simulink model "ES200A_CurrMeas"  (R2013b)
settings: Solver=FixedStepDiscrete  SolverMode=SingleTasking  StartTime=0.0  StopTime=1  FixedStep=0.000125  RelTol=1e-3
undefined symbols (not defined in the file): ARCHGLBPRM_2PI_ULS_F32, CurrMeasEolGainMax, CurrMeasEolGainMin, CurrMeasEolGainNrOfSample, CurrMeasEolGainNumer, CurrMeasEolMaxMotVel, CurrMeasEolOffsHiBrdgVltgMin, CurrMeasEolOffsHiCmuOffs, CurrMeasEolOffsLoCmuOffs, CurrMeasEolOffsMax, CurrMeasEolOffsMin, CurrMeasEolOffsNrOfSample, CurrMeasEolTranCntrThd, CurrMeasMinRqrdPhaOnTi, CurrMeasMotAgCompuDly, CurrMeasMotCurrAdcVlyWrmIninMax, CurrMeasMotCurrAdcVlyWrmIninMin, CurrMeasNtc0x05DFailStep, CurrMeasNtc0x05DPassStep, CurrMeasNtc0x06DFailStep, CurrMeasNtc0x06DPassStep, DEGREES30_MOTRAD_F32, DIFOFFSRNGCHKMAX_VOLT_F32, ELECGLBPRM_IVTRCNT_CNT_U08, ELECGLBPRM_STRTUPSTCURRMEASWRMININTESTSTRT_CNT_U08, FLTINJ_CURRMEAS_MOTCURRCORRDA, FLTINJ_CURRMEAS_MOTCURRCORRDD, FLTINJ_CURRMEAS_TESTOK, MAXCURRCORRD_AMPR_F32, PhaABCMeasdOutOfRng, PhaDEFMeasOutOfRng, SysGlbPrmMotPoleCnt
libraries: simulink x10, FixdToFloat x1
(part 3 of 7)

== system ES200A_CurrMeas/CurrMeas/CurrMeasGainWrReq ==
  CurrMeasMotCurrGainA_ArgIn : Inport  RequirementInfo={} %GIDa_c425d1ca_be7a_40e5_bba5_162e843ab10f  OutDataTypeStr=single
  CurrMeasMotCurrGainB_ArgIn : Inport  RequirementInfo={} %GIDa_bd7d1dd6_00d8_4c0e_b958_cd79b1c62016  Port=2  OutDataTypeStr=single
  CurrMeasMotCurrGainC_ArgIn : Inport  RequirementInfo={} %GIDa_442e802f_e2c7_406d_b1fc_b8f70d0353c6  Port=3  OutDataTypeStr=single
  CurrMeasMotCurrGainD_ArgIn : Inport  RequirementInfo={} %GIDa_a6de7fab_9a7f_4a18_932a_688a0ad19497  Port=4  OutDataTypeStr=single
  CurrMeasMotCurrGainE_ArgIn : Inport  RequirementInfo={} %GIDa_58241980_a2a0_46cb_8faf_4af881b5bc84  Port=5  OutDataTypeStr=single
  CurrMeasMotCurrGainF_ArgIn : Inport  RequirementInfo={} %GIDa_7c5d0880_7e38_46fb_95a6_ac4fe6cd7a27  Port=6  OutDataTypeStr=single
  function : TriggerPort
  Constant1 : Constant  Value=CurrMeasEolGainMax  OutDataTypeStr=single
  Constant3 : Constant  Value=CurrMeasEolGainMin  OutDataTypeStr=single
  CopyRight2 : Subsystem  Description=|  mask(Copyright Information){none=on}
      | Copyright info block.                                               
      |                                                                     
      | Place copyright information at the top of every subsystem in design.
      mask prompts: none "No parameters"
      mask help: Place copyright information at the top of every subsystem in design.
      mask Display:
      | NxtrConf = 'Nexteer Confidential';
      | 
      | sys = bdroot; %handle for the current model ("system")
      | first = get_param(sys,'Created');
      | first = first(end-3:end);  %year is last four digits
      | 
      | last = get_param(sys,'LastModifiedDate');
      | if isempty(last)
      |     last = datestr(now,'yyyy');
      | else
      |     last = last(end-3:end);
      | end
      | 
      | if strcmp(first,last)
      |     fprintf('%s -- Copyright %s Nexteer',NxtrConf,first)
      | else
      |     fprintf('%s -- %s%s- %s Nexteer',NxtrConf,char(169),first,last)
      | end
  IF : Subsystem  RequirementInfo={'linktype_rmi_doors' '000089bc (/ESG Group/FDD Module Requirements/EA4 Specific/ES200A_CurrMeas)' '#ES200A_291' 'true' 'REQ: ES200A_291' '' } %GIDa_4876ff6b_f5fc_4b95_bbc0_660fa9cc47c9  TreatAsAtomicUnit=on
  If1 : If  RequirementInfo={'linktype_rmi_doors' '000089bc (/ESG Group/FDD Module Requirements/EA4 Specific/ES200A_CurrMeas)' '#ES200A_291' 'true' 'REQ: ES200A_291' '' } %GIDa_99201fd8_db84_4d56_a868_77c34be46a9e  NumInputs=8  IfExpression=(u1 <= u3 & u3 <= u2) & (u1 <= u4 & u4 <= u2) & (u1 <= u5 & u5 <= u2) & (u1 <= u6 & u6 <= u2) & (u1 <= u7 & u7 <= u2) & (u1 <= u8 & u8 <= u2)
  Merge : Merge
  "else " : Subsystem  TreatAsAtomicUnit=on
  CurrMeasGainWrReqSts : Outport  RequirementInfo={} %GIDa_00298d30_c602_4e54_ac9c_fe9e46cb7e08
  wires:
  If1/1 -> IF/Action
  Constant3/1 -> If1/1
  Constant1/1 -> If1/2
  CurrMeasMotCurrGainC_ArgIn/1 -> IF/3(CurrMeasMotCurrGainC_ArgIn), If1/5  "CurrMeasMotCurrGainC_ArgIn"
  CurrMeasMotCurrGainD_ArgIn/1 -> IF/4(CurrMeasMotCurrGainD_ArgIn), If1/6  "CurrMeasMotCurrGainD_ArgIn"
  CurrMeasMotCurrGainB_ArgIn/1 -> IF/2(CurrMeasMotCurrGainB_ArgIn), If1/4  "CurrMeasMotCurrGainB_ArgIn"
  CurrMeasMotCurrGainE_ArgIn/1 -> IF/5(CurrMeasMotCurrGainE_ArgIn), If1/7  "CurrMeasMotCurrGainE_ArgIn"
  CurrMeasMotCurrGainA_ArgIn/1 -> IF/1(CurrMeasMotCurrGainA_ArgIn), If1/3  "CurrMeasMotCurrGainA_ArgIn"
  CurrMeasMotCurrGainF_ArgIn/1 -> IF/6(CurrMeasMotCurrGainF_ArgIn), If1/8  "CurrMeasMotCurrGainF_ArgIn"
  If1/2 -> "else "/Action
  Merge/1 -> CurrMeasGainWrReqSts/1
  "else "/1(CurrMeasGainWrReqSts) -> Merge/1
  IF/1(CurrMeasGainWrReqSts) -> Merge/2

== system ES200A_CurrMeas/CurrMeas/CurrMeasInit1 ==
  CurrMeasEolOffsHiBrdgVltgMin : Inport
  Trigger : TriggerPort  TriggerType=function-call  PortDimensions=1
  CopyRight2 : Subsystem  Description=|  mask(Copyright Information){none=on}
      | Copyright info block.                                               
      |                                                                     
      | Place copyright information at the top of every subsystem in design.
      mask prompts: none "No parameters"
      mask help: Place copyright information at the top of every subsystem in design.
      mask Display:
      | NxtrConf = 'Nexteer Confidential';
      | 
      | sys = bdroot; %handle for the current model ("system")
      | first = get_param(sys,'Created');
      | first = first(end-3:end);  %year is last four digits
      | 
      | last = get_param(sys,'LastModifiedDate');
      | if isempty(last)
      |     last = datestr(now,'yyyy');
      | else
      |     last = last(end-3:end);
      | end
      | 
      | if strcmp(first,last)
      |     fprintf('%s -- Copyright %s Nexteer',NxtrConf,first)
      | else
      |     fprintf('%s -- %s%s- %s Nexteer',NxtrConf,char(169),first,last)
      | end
  CurrMeasEolOffsCalSet : DataStoreRead  RequirementInfo={'linktype_rmi_doors' '000089bc (/ESG Group/FDD Module Requirements/EA4 Specific/ES200A_CurrMeas)' '#ES200A_280' 'true' 'REQ: ES200A_280' '' } %GIDa_5b13b3a8_fa13_45cc_ae87_baf34a1014a6  DataStoreName=CurrMeasEolOffsCalSet  DataStoreElements=CurrMeasEolOffsCalSet.CurrMeasMotCurrEolOffsDifA#CurrMeasEolOffsCalSet.CurrMeasMotCurrEolOffsDifB#CurrMeasEolOffsCalSet.CurrMeasMotCurrEolOffsDifC#CurrMeasEolOffsCalSet.CurrMeasEolOffsHiBrdgVltg#CurrMeasEolOffsCalSet.CurrMeasMotCurrEolOffsDifD#CurrMeasEolOffsCalSet.CurrMeasMotCurrEolOffsDifE#CurrMeasEolOffsCalSet.CurrMeasMotCurrEolOffsDifF
  If : If  NumInputs=2  IfExpression=u1>u2
  If Action Subsystem : Subsystem  TreatAsAtomicUnit=on
  If Action Subsystem1 : Subsystem  TreatAsAtomicUnit=on
  Merge{1..6} (6 alike) : Merge
  MotCurrOffsDeltaA : Outport
  MotCurrOffsDeltaB : Outport  Port=2
  MotCurrOffsDeltaC : Outport  Port=3
  MotCurrOffsDeltaD : Outport  Port=4
  MotCurrOffsDeltaE : Outport  Port=5
  MotCurrOffsDeltaF : Outport  Port=6
  wires:
  CurrMeasEolOffsHiBrdgVltgMin/1 -> If/2
  If/1 -> If Action Subsystem/Action
  If/2 -> If Action Subsystem1/Action
  If Action Subsystem/1(MotCurrOffsDeltaA) -> Merge1/1
  If Action Subsystem/2(MotCurrOffsDeltaB) -> Merge2/1
  If Action Subsystem/3(MotCurrOffsDeltaC) -> Merge3/1
  If Action Subsystem/4(MotCurrOffsDeltaD) -> Merge4/1
  If Action Subsystem/5(MotCurrOffsDeltaE) -> Merge5/1
  If Action Subsystem/6(MotCurrOffsDeltaF) -> Merge6/1
  If Action Subsystem1/1(MotCurrOffsDeltaA) -> Merge1/2
  If Action Subsystem1/2(MotCurrOffsDeltaB) -> Merge2/2
  If Action Subsystem1/3(MotCurrOffsDeltaC) -> Merge3/2
  If Action Subsystem1/4(MotCurrOffsDeltaD) -> Merge4/2
  If Action Subsystem1/5(MotCurrOffsDeltaE) -> Merge5/2
  If Action Subsystem1/6(MotCurrOffsDeltaF) -> Merge6/2
  Merge1/1 -> MotCurrOffsDeltaA/1
  Merge2/1 -> MotCurrOffsDeltaB/1
  Merge3/1 -> MotCurrOffsDeltaC/1
  Merge4/1 -> MotCurrOffsDeltaD/1
  Merge5/1 -> MotCurrOffsDeltaE/1
  Merge6/1 -> MotCurrOffsDeltaF/1
  CurrMeasEolOffsCalSet/5 -> If Action Subsystem/5(MotCurrEolOffsDifD)
  CurrMeasEolOffsCalSet/3 -> If Action Subsystem/3(MotCurrEolOffsDifC)
  CurrMeasEolOffsCalSet/6 -> If Action Subsystem/6(MotCurrEolOffsDifE)
  CurrMeasEolOffsCalSet/1 -> If Action Subsystem/1(MotCurrEolOffsDifA)
  CurrMeasEolOffsCalSet/2 -> If Action Subsystem/2(MotCurrEolOffsDifB)
  CurrMeasEolOffsCalSet/7 -> If Action Subsystem/7(MotCurrEolOffsDifF)
  CurrMeasEolOffsCalSet/4 -> If/1, If Action Subsystem/4(CurrMeasEolOffsHiBrdgVltg)

== system ES200A_CurrMeas/CurrMeas/CurrMeasOffsReadReq ==
  function : TriggerPort
  CopyRight2 : Subsystem  Description=|  mask(Copyright Information){none=on}
      | Copyright info block.                                               
      |                                                                     
      | Place copyright information at the top of every subsystem in design.
      mask prompts: none "No parameters"
      mask help: Place copyright information at the top of every subsystem in design.
      mask Display:
      | NxtrConf = 'Nexteer Confidential';
      | 
      | sys = bdroot; %handle for the current model ("system")
      | first = get_param(sys,'Created');
      | first = first(end-3:end);  %year is last four digits
      | 
      | last = get_param(sys,'LastModifiedDate');
      | if isempty(last)
      |     last = datestr(now,'yyyy');
      | else
      |     last = last(end-3:end);
      | end
      | 
      | if strcmp(first,last)
      |     fprintf('%s -- Copyright %s Nexteer',NxtrConf,first)
      | else
      |     fprintf('%s -- %s%s- %s Nexteer',NxtrConf,char(169),first,last)
      | end
  CurrMeasEolOffsCalSet : DataStoreRead  RequirementInfo={'linktype_rmi_doors' '000089bc (/ESG Group/FDD Module Requirements/EA4 Specific/ES200A_CurrMeas)' '#ES200A_280' 'true' 'REQ: ES200A_280' '' } %GIDa_8cba0bc8_e323_4e1f_8e86_73dafe0bba1d  DataStoreName=CurrMeasEolOffsCalSet  DataStoreElements=CurrMeasEolOffsCalSet.CurrMeasEolOffsHiBrdgVltg#CurrMeasEolOffsCalSet.CurrMeasMotCurrEolOffsDifA#CurrMeasEolOffsCalSet.CurrMeasMotCurrEolOffsDifB#CurrMeasEolOffsCalSet.CurrMeasMotCurrEolOffsDifC#CurrMeasEolOffsCalSet.CurrMeasMotCurrEolOffsDifD#CurrMeasEolOffsCalSet.CurrMeasMotCurrEolOffsDifE#CurrMeasEolOffsCalSet.CurrMeasMotCurrEolOffsDifF#CurrMeasEolOffsCalSet.CurrMeasMotCurrOffsLoAvrgA#CurrMeasEolOffsCalSet.CurrMeasMotCurrOffsLoAvrgB#CurrMeasEolOffsCalSet.CurrMeasMotCurrOffsLoAvrgC#CurrMeasEolOffsCalSet.CurrMeasMotCurrOffsLoAvrgD#CurrMeasEolOffsCalSet.CurrMeasMotCurrOffsLoAvrgE#CurrMeasEolOffsCalSet.CurrMeasMotCurrOffsLoAvrgF
  CurrMeasEolOffsHiBrdgVltg_ArgOut : Outport  RequirementInfo={} %GIDa_c2b0fe9d_3793_43b9_8623_9e15e29718c9
  CurrMeasMotCurrOffsDifA_ArgOut : Outport  RequirementInfo={} %GIDa_06880cd0_b3c9_4dac_a20b_1d769ce6ab3e  Port=2
  CurrMeasMotCurrOffsDifB_ArgOut : Outport  RequirementInfo={} %GIDa_89879a61_0bc4_4d01_9a03_1b0943ab4d4d  Port=3
  CurrMeasMotCurrOffsDifC_ArgOut : Outport  RequirementInfo={} %GIDa_a1432bf3_c07e_4e99_b270_4232122d4772  Port=4
  CurrMeasMotCurrOffsDifD_ArgOut : Outport  RequirementInfo={} %GIDa_3df17fd6_11a6_4a3b_a21f_0f2b4386103a  Port=5
  CurrMeasMotCurrOffsDifE_ArgOut : Outport  RequirementInfo={} %GIDa_8531bc1c_851e_4a5c_bd1a_ff758ac49903  Port=6
  CurrMeasMotCurrOffsDifF_ArgOut : Outport  RequirementInfo={} %GIDa_d9d2e87e_a616_4443_9719_46d0ee8ea0d2  Port=7
  CurrMeasMotCurrOffsLoAvrgA_ArgOut : Outport  RequirementInfo={} %GIDa_c5194a62_6435_4295_b125_fb72e5f95c25  Port=8
  CurrMeasMotCurrOffsLoAvrgB_ArgOut : Outport  RequirementInfo={} %GIDa_76f08b3f_5cc7_46f2_a183_091f4f2205e6  Port=9
  CurrMeasMotCurrOffsLoAvrgC_ArgOut : Outport  RequirementInfo={} %GIDa_b1bbc18a_9d6a_4672_bdc3_0bccd18a5fef  Port=10
  CurrMeasMotCurrOffsLoAvrgD_ArgOut : Outport  RequirementInfo={} %GIDa_3f8d0b0a_e576_41bf_81a1_80b77bc69872  Port=11
  CurrMeasMotCurrOffsLoAvrgE_ArgOut : Outport  RequirementInfo={} %GIDa_06d47c59_3406_4ddb_96f7_958a6ee8ee04  Port=12
  CurrMeasMotCurrOffsLoAvrgF_ArgOut : Outport  RequirementInfo={} %GIDa_8b869263_e1b4_42a0_8921_d65f6bf7b80b  Port=13
  wires:
  CurrMeasEolOffsCalSet/1 -> CurrMeasEolOffsHiBrdgVltg_ArgOut/1
  CurrMeasEolOffsCalSet/2 -> CurrMeasMotCurrOffsDifA_ArgOut/1
  CurrMeasEolOffsCalSet/3 -> CurrMeasMotCurrOffsDifB_ArgOut/1
  CurrMeasEolOffsCalSet/4 -> CurrMeasMotCurrOffsDifC_ArgOut/1
  CurrMeasEolOffsCalSet/5 -> CurrMeasMotCurrOffsDifD_ArgOut/1
  CurrMeasEolOffsCalSet/6 -> CurrMeasMotCurrOffsDifE_ArgOut/1
  CurrMeasEolOffsCalSet/7 -> CurrMeasMotCurrOffsDifF_ArgOut/1
  CurrMeasEolOffsCalSet/8 -> CurrMeasMotCurrOffsLoAvrgA_ArgOut/1
  CurrMeasEolOffsCalSet/9 -> CurrMeasMotCurrOffsLoAvrgB_ArgOut/1
  CurrMeasEolOffsCalSet/10 -> CurrMeasMotCurrOffsLoAvrgC_ArgOut/1
  CurrMeasEolOffsCalSet/11 -> CurrMeasMotCurrOffsLoAvrgD_ArgOut/1
  CurrMeasEolOffsCalSet/12 -> CurrMeasMotCurrOffsLoAvrgE_ArgOut/1
  CurrMeasEolOffsCalSet/13 -> CurrMeasMotCurrOffsLoAvrgF_ArgOut/1

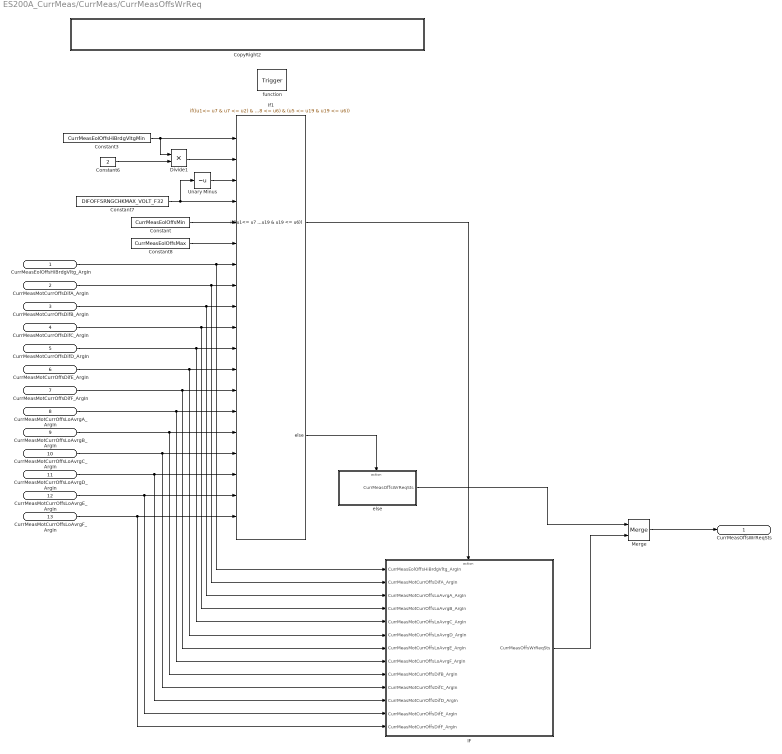
== system ES200A_CurrMeas/CurrMeas/CurrMeasOffsWrReq ==
  CurrMeasEolOffsHiBrdgVltg_ArgIn : Inport  RequirementInfo={} %GIDa_20319714_70ba_40b8_83d5_5be49dcbe6c0  OutDataTypeStr=single
  CurrMeasMotCurrOffsDifA_ArgIn : Inport  RequirementInfo={} %GIDa_567da3a1_0d48_4934_8feb_e936b086fb7e  Port=2  OutDataTypeStr=single
  CurrMeasMotCurrOffsDifB_ArgIn : Inport  RequirementInfo={} %GIDa_d0ed0aa3_f35f_4142_b108_d1399608bd37  Port=3  OutDataTypeStr=single
  CurrMeasMotCurrOffsDifC_ArgIn : Inport  RequirementInfo={} %GIDa_333f9d57_9630_4d9a_bf0a_758004fd24d5  Port=4  OutDataTypeStr=single
  CurrMeasMotCurrOffsDifD_ArgIn : Inport  RequirementInfo={} %GIDa_75702a95_bde2_4d36_99b5_54163b4c7153  Port=5  OutDataTypeStr=single
  CurrMeasMotCurrOffsDifE_ArgIn : Inport  RequirementInfo={} %GIDa_d5c11ab6_7fa1_4a01_9aa2_8e70eb92dca0  Port=6  OutDataTypeStr=single
  CurrMeasMotCurrOffsDifF_ArgIn : Inport  RequirementInfo={} %GIDa_93b2894a_d1d3_46df_b4ef_6d97a088df41  Port=7  OutDataTypeStr=single
  CurrMeasMotCurrOffsLoAvrgA_ArgIn : Inport  RequirementInfo={} %GIDa_d3fc1696_9b01_4bfe_ae5b_43ed0baf9797  Port=8  OutDataTypeStr=single
  CurrMeasMotCurrOffsLoAvrgB_ArgIn : Inport  RequirementInfo={} %GIDa_e3286a61_69ab_4ddc_b4c3_7297f20485dd  Port=9  OutDataTypeStr=single
  CurrMeasMotCurrOffsLoAvrgC_ArgIn : Inport  RequirementInfo={} %GIDa_d0fb0236_0795_4629_a145_caa3ab5bd346  Port=10  OutDataTypeStr=single
  CurrMeasMotCurrOffsLoAvrgD_ArgIn : Inport  RequirementInfo={} %GIDa_8377999d_f727_4278_a09a_19b59b7325e4  Port=11  OutDataTypeStr=single
  CurrMeasMotCurrOffsLoAvrgE_ArgIn : Inport  RequirementInfo={} %GIDa_308508b2_c858_4477_ae29_a4055a9a0165  Port=12  OutDataTypeStr=single
  CurrMeasMotCurrOffsLoAvrgF_ArgIn : Inport  RequirementInfo={} %GIDa_00179445_133e_4a7c_829d_b4552183115d  Port=13  OutDataTypeStr=single
  function : TriggerPort
  Constant : Constant  Value=CurrMeasEolOffsMin
  Constant3 : Constant  Value=CurrMeasEolOffsHiBrdgVltgMin  OutDataTypeStr=single
  Constant6 : Constant  Value=2  OutDataTypeStr=single
  Constant7 : Constant  Value=DIFOFFSRNGCHKMAX_VOLT_F32  OutDataTypeStr=single
  Constant8 : Constant  Value=CurrMeasEolOffsMax
  CopyRight2 : Subsystem  Description=|  mask(Copyright Information){none=on}
      | Copyright info block.                                               
      |                                                                     
      | Place copyright information at the top of every subsystem in design.
      mask prompts: none "No parameters"
      mask help: Place copyright information at the top of every subsystem in design.
      mask Display:
      | NxtrConf = 'Nexteer Confidential';
      | 
      | sys = bdroot; %handle for the current model ("system")
      | first = get_param(sys,'Created');
      | first = first(end-3:end);  %year is last four digits
      | 
      | last = get_param(sys,'LastModifiedDate');
      | if isempty(last)
      |     last = datestr(now,'yyyy');
      | else
      |     last = last(end-3:end);
      | end
      | 
      | if strcmp(first,last)
      |     fprintf('%s -- Copyright %s Nexteer',NxtrConf,first)
      | else
      |     fprintf('%s -- %s%s- %s Nexteer',NxtrConf,char(169),first,last)
      | end
  Divide1 : Product  Inputs=**  OutDataTypeStr=single
  IF : Subsystem  RequirementInfo={'linktype_rmi_doors' '000089bc (/ESG Group/FDD Module Requirements/EA4 Specific/ES200A_CurrMeas)' '#ES200A_280' 'true' 'REQ: ES200A_280' '' } %GIDa_94ca970e_96f2_476d_8160_5cb99576e311  TreatAsAtomicUnit=on
  If1 : If  RequirementInfo={'linktype_rmi_doors' '000089bc (/ESG Group/FDD Module Requirements/EA4 Specific/ES200A_CurrMeas)' '#ES200A_280' 'true' 'REQ: ES200A_280' '' } %GIDa_9a24cfae_c3f3_4b93_a488_aa733d7ab090  NumInputs=19  IfExpression=(u1<= u7 & u7 <= u2) & (u3 <= u8 & u8 <= u4) & (u3 <= u9 & u9 <= u4) & (u3 <= u10 & u10 < u4) & (u3 <= u11 & u11 <= u4) & (u3 <= u12 & u12 <= u4) & (u3 <= u13 & u13 <= u4) & (u5 <= u14 & u14 <= u6) & (u5 <= u15 & u15 <= u6) & (u5 <= u16 & u16 <= u6) & (u5 <= u17 & u17 <= u6) & (u5 <= u18 & u18 <= u6) & (u5 <= u19 & u19 <= u6)
  Merge : Merge
  Unary Minus : UnaryMinus
  "else " : Subsystem  TreatAsAtomicUnit=on
  CurrMeasOffsWrReqSts : Outport  RequirementInfo={} %GIDa_e38a5dae_03c2_4788_8854_754d30bf24dd
  wires:
  Constant3/1 -> If1/1, Divide1/1
  Constant6/1 -> Divide1/2
  Unary Minus/1 -> If1/3
  Constant7/1 -> Unary Minus/1, If1/4
  Constant8/1 -> If1/6
  Constant/1 -> If1/5
  CurrMeasEolOffsHiBrdgVltg_ArgIn/1 -> IF/1(CurrMeasEolOffsHiBrdgVltg_ArgIn), If1/7
  CurrMeasMotCurrOffsDifA_ArgIn/1 -> IF/2(CurrMeasMotCurrOffsDifA_ArgIn), If1/8
  CurrMeasMotCurrOffsDifB_ArgIn/1 -> IF/3(CurrMeasMotCurrOffsLoAvrgA_ArgIn), If1/9
  CurrMeasMotCurrOffsDifC_ArgIn/1 -> IF/4(CurrMeasMotCurrOffsLoAvrgB_ArgIn), If1/10
  CurrMeasMotCurrOffsDifD_ArgIn/1 -> IF/5(CurrMeasMotCurrOffsLoAvrgC_ArgIn), If1/11
  CurrMeasMotCurrOffsDifE_ArgIn/1 -> IF/6(CurrMeasMotCurrOffsLoAvrgD_ArgIn), If1/12
  CurrMeasMotCurrOffsLoAvrgA_ArgIn/1 -> IF/8(CurrMeasMotCurrOffsLoAvrgF_ArgIn), If1/14
  CurrMeasMotCurrOffsLoAvrgB_ArgIn/1 -> IF/9(CurrMeasMotCurrOffsDifB_ArgIn), If1/15
  CurrMeasMotCurrOffsLoAvrgE_ArgIn/1 -> IF/12(CurrMeasMotCurrOffsDifE_ArgIn), If1/18
  CurrMeasMotCurrOffsLoAvrgF_ArgIn/1 -> IF/13(CurrMeasMotCurrOffsDifF_ArgIn), If1/19
  CurrMeasMotCurrOffsLoAvrgC_ArgIn/1 -> IF/10(CurrMeasMotCurrOffsDifC_ArgIn), If1/16
  If1/1 -> IF/Action
  CurrMeasMotCurrOffsDifF_ArgIn/1 -> IF/7(CurrMeasMotCurrOffsLoAvrgE_ArgIn), If1/13
  CurrMeasMotCurrOffsLoAvrgD_ArgIn/1 -> IF/11(CurrMeasMotCurrOffsDifD_ArgIn), If1/17
  If1/2 -> "else "/Action
  Divide1/1 -> If1/2
  Merge/1 -> CurrMeasOffsWrReqSts/1
  "else "/1(CurrMeasOffsWrReqSts) -> Merge/1
  IF/1(CurrMeasOffsWrReqSts) -> Merge/2

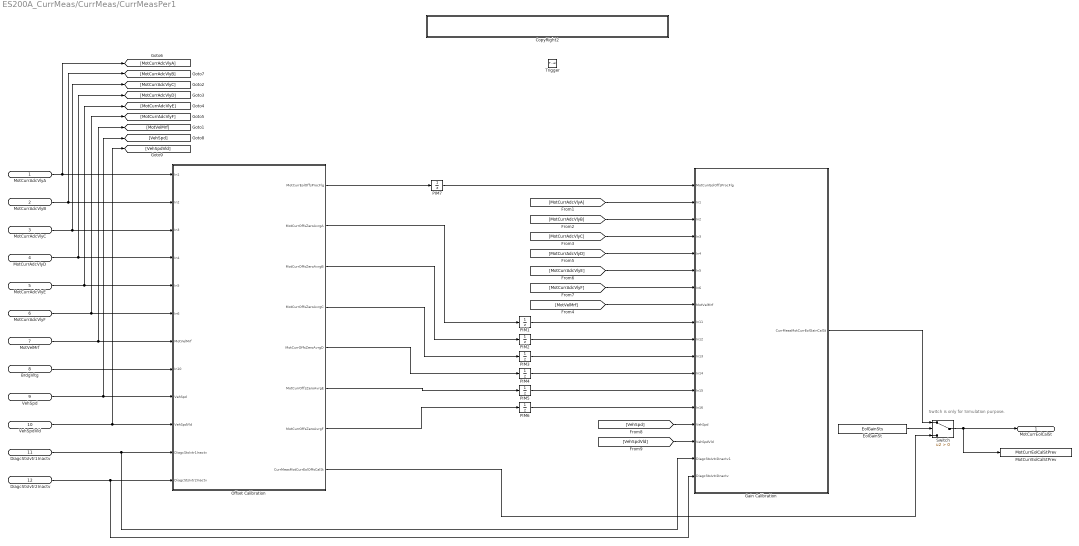
== system ES200A_CurrMeas/CurrMeas/CurrMeasPer1 ==
  note: Switch is only for Simulation purpose.
  MotCurrAdcVlyA : Inport  RequirementInfo={} %GIDa_d6fdc2a5_c36f_4862_a3e7_4b336023a3c4  OutDataTypeStr=single
  MotCurrAdcVlyB : Inport  RequirementInfo={} %GIDa_329e32be_6008_45fd_bd72_340d7ae8c1b5  Port=2  OutDataTypeStr=single
  MotCurrAdcVlyC : Inport  RequirementInfo={} %GIDa_746c9616_e976_40d7_b54a_823dc364fe71  Port=3  OutDataTypeStr=single
  MotCurrAdcVlyD : Inport  RequirementInfo={} %GIDa_4b06763f_6209_4b7f_9565_5c5d2daca03a  Port=4  OutDataTypeStr=single
  MotCurrAdcVlyE : Inport  RequirementInfo={} %GIDa_3a5b9e65_aa66_45a4_8818_13580434b978  Port=5  OutDataTypeStr=single
  MotCurrAdcVlyF : Inport  RequirementInfo={} %GIDa_3a4efe1c_5ef6_4746_95ad_6493d8eca6d1  Port=6  OutDataTypeStr=single
  MotVelMrf : Inport  RequirementInfo={} %GIDa_3549e207_a5ba_4370_a041_76429f88a9dd  Port=7  OutDataTypeStr=single
  BrdgVltg : Inport  RequirementInfo={} %GIDa_3ee59834_071a_42af_a764_5aee71a021cf  Port=8  OutDataTypeStr=single
  VehSpd : Inport  RequirementInfo={} %GIDa_3dad792b_6867_498d_8cf5_08b87633e71b  Port=9
  VehSpdVld : Inport  RequirementInfo={} %GIDa_79ad4a0e_1634_487e_a0d4_030cd7a6c3f9  Port=10
  DiagcStsIvtr1Inactv : Inport  RequirementInfo={} %GIDa_c8c114ff_24fe_44c5_88f9_1823b0535249  Port=11
  DiagcStsIvtr2Inactv : Inport  RequirementInfo={} %GIDa_6fd709e7_73cf_4f38_ab69_3c4606ea6b91  Port=12
  Trigger : TriggerPort  TriggerType=function-call  PortDimensions=1
  CopyRight2 : Subsystem  Description=|  mask(Copyright Information){none=on}
      | Copyright info block.                                               
      |                                                                     
      | Place copyright information at the top of every subsystem in design.
      mask prompts: none "No parameters"
      mask help: Place copyright information at the top of every subsystem in design.
      mask Display:
      | NxtrConf = 'Nexteer Confidential';
      | 
      | sys = bdroot; %handle for the current model ("system")
      | first = get_param(sys,'Created');
      | first = first(end-3:end);  %year is last four digits
      | 
      | last = get_param(sys,'LastModifiedDate');
      | if isempty(last)
      |     last = datestr(now,'yyyy');
      | else
      |     last = last(end-3:end);
      | end
      | 
      | if strcmp(first,last)
      |     fprintf('%s -- Copyright %s Nexteer',NxtrConf,first)
      | else
      |     fprintf('%s -- %s%s- %s Nexteer',NxtrConf,char(169),first,last)
      | end
  EolGainSt : DataStoreRead  DataStoreName=EolGainSts
  Gain Calibration : Subsystem  RequirementInfo={} %GIDa_dc55cc08_00d5_4d2c_9161_2782955335b3
  MotCurrEolCalStPrev : DataStoreWrite  RequirementInfo={} %GIDa_5bd07b1c_86e4_46fd_afdc_b357d0f0069c  DataStoreName=MotCurrEolCalStPrev  DataStoreElements=MotCurrEolCalStPrev
  Offset Calibration : Subsystem  RequirementInfo={} %GIDa_31f7e6d5_3bce_40cc_a784_8fd3d5abd669
  PIM1 : UnitDelay  SampleTime=-1  StateName=MotCurrOffsZeroAvrgA  StateMustResolveToSignalObject=on
      settings: AttributesFormatString=%<StateName>
  PIM2 : UnitDelay  SampleTime=-1  StateName=MotCurrOffsZeroAvrgB  StateMustResolveToSignalObject=on
      settings: AttributesFormatString=%<StateName>
  PIM3 : UnitDelay  SampleTime=-1  StateName=MotCurrOffsZeroAvrgC  StateMustResolveToSignalObject=on
      settings: AttributesFormatString=%<StateName>
  PIM4 : UnitDelay  SampleTime=-1  StateName=MotCurrOffsZeroAvrgD  StateMustResolveToSignalObject=on
      settings: AttributesFormatString=%<StateName>
  PIM5 : UnitDelay  SampleTime=-1  StateName=MotCurrOffsZeroAvrgE  StateMustResolveToSignalObject=on
      settings: AttributesFormatString=%<StateName>
  PIM6 : UnitDelay  SampleTime=-1  StateName=MotCurrOffsZeroAvrgF  StateMustResolveToSignalObject=on
      settings: AttributesFormatString=%<StateName>
  PIM7 : UnitDelay  SampleTime=-1  StateName=MotCurrEolOffsProcFlg  StateMustResolveToSignalObject=on
      settings: AttributesFormatString=%<StateName>
  Switch : Switch  Criteria=u2 > Threshold  OutDataTypeStr=Inherit: Inherit via back propagation
  MotCurrEolCalSt : Outport  RequirementInfo={} %GIDa_bd1a9dea_c496_413a_aa00_f3bf38f71498
  wires:
  Offset Calibration/2(MotCurrOffsZeroAvrgA) -> PIM1/1
  Offset Calibration/3(MotCurrOffsZeroAvrgB) -> PIM2/1
  Offset Calibration/4(MotCurrOffsZeroAvrgC) -> PIM3/1
  Offset Calibration/5(MotCurrOffsZeroAvrgD) -> PIM4/1
  Offset Calibration/6(MotCurrOffsZeroAvrgE) -> PIM5/1
  Offset Calibration/7(MotCurrOffsZeroAvrgF) -> PIM6/1
  Offset Calibration/1("MotCurrEolOffsProcFlg ") -> PIM7/1
  [VehSpd] -> Gain Calibration/15(VehSpd)
  [VehSpdVld] -> Gain Calibration/16(VehSpdVld)
  MotCurrAdcVlyA/1 -> Offset Calibration/1(In1), [MotCurrAdcVlyA]
  MotCurrAdcVlyC/1 -> [MotCurrAdcVlyC], Offset Calibration/3(In3)
  MotCurrAdcVlyE/1 -> [MotCurrAdcVlyE], Offset Calibration/5(In5)
  MotCurrAdcVlyD/1 -> [MotCurrAdcVlyD], Offset Calibration/4(In4)
  MotCurrAdcVlyB/1 -> [MotCurrAdcVlyB], Offset Calibration/2(In2)
  VehSpd/1 -> [VehSpd], Offset Calibration/9(VehSpd)
  BrdgVltg/1 -> Offset Calibration/8(In10)
  MotCurrAdcVlyF/1 -> [MotCurrAdcVlyF], Offset Calibration/6(In6)
  VehSpdVld/1 -> [VehSpdVld], Offset Calibration/10(VehSpdVld)
  MotVelMrf/1 -> [MotVelMrf], Offset Calibration/7(MotVelMrf)
  [MotCurrAdcVlyF] -> Gain Calibration/7(In6)
  [MotCurrAdcVlyB] -> Gain Calibration/3(In2)
  [MotCurrAdcVlyD] -> Gain Calibration/5(In4)
  [MotCurrAdcVlyE] -> Gain Calibration/6(In5)
  [MotCurrAdcVlyC] -> Gain Calibration/4(In3)
  [MotCurrAdcVlyA] -> Gain Calibration/2(In1)
  [MotVelMrf] -> Gain Calibration/8(MotVelMrf)
  PIM1/1 -> Gain Calibration/9(In11)
  PIM2/1 -> Gain Calibration/10(In12)
  PIM3/1 -> Gain Calibration/11(In13)
  PIM4/1 -> Gain Calibration/12(In14)
  PIM5/1 -> Gain Calibration/13(In15)
  PIM6/1 -> Gain Calibration/14(In16)
  PIM7/1 -> Gain Calibration/1(MotCurrEolOffsProcFlg)
  DiagcStsIvtr2Inactv/1 -> Gain Calibration/18(DiagcStsIvtr2Inactv), Offset Calibration/12(DiagcStsIvtr2Inactv)
  DiagcStsIvtr1Inactv/1 -> Gain Calibration/17(DiagcStsIvtr2Inactv1), Offset Calibration/11(DiagcStsIvtr1Inactv)
  Gain Calibration/1(CurrMeasMotCurrEolGainCalSt) -> Switch/1
  Offset Calibration/8(CurrMeasMotCurrEolOffsCalSt) -> Switch/3
  Switch/1 -> MotCurrEolCalStPrev/1, MotCurrEolCalSt/1
  EolGainSt/1 -> Switch/2

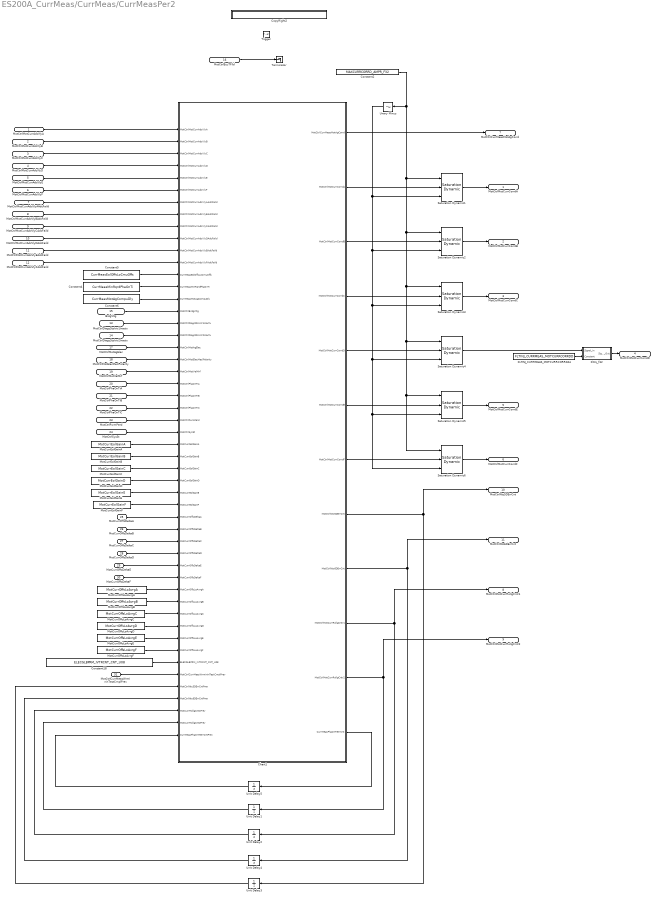
== system ES200A_CurrMeas/CurrMeas/CurrMeasPer2 ==
  MotCtrlMotCurrAdcVlyA : Inport  RequirementInfo={} %GIDa_51523d33_6191_4b88_8694_817dc9ded571
  MotCtrlMotCurrAdcVlyB : Inport  RequirementInfo={} %GIDa_1328ae42_ae96_4bf4_89b7_7635d71eb55f  Port=2
  MotCtrlMotCurrAdcVlyC : Inport  RequirementInfo={} %GIDa_141aa39a_2219_4c7a_8648_7879c9127c56  Port=3
  MotCtrlMotCurrAdcVlyD : Inport  RequirementInfo={} %GIDa_0bb8dbbc_c7c5_4117_b4a1_ced2a35897c9  Port=4
  MotCtrlMotCurrAdcVlyE : Inport  RequirementInfo={} %GIDa_e7be49ef_22f9_4690_b020_08185c31c438  Port=5
  MotCtrlMotCurrAdcVlyF : Inport  RequirementInfo={} %GIDa_885c6b45_efc1_4125_8826_e1fe2f9bfc98  Port=6
  MotCtrlMotCurrAdcVlyAAdcFaild : Inport  RequirementInfo={} %GIDa_d667bfad_9ccb_4ad0_ab64_59c5adeb3cfc  Port=7
  MotCtrlMotCurrAdcVlyBAdcFaild : Inport  RequirementInfo={} %GIDa_614f9520_457f_4a4d_a608_e6a9d7384c30  Port=8
  MotCtrlMotCurrAdcVlyCAdcFaild : Inport  RequirementInfo={} %GIDa_26dea516_d730_426b_b0f7_aef164a4b4a7  Port=9
  MotCtrlMotCurrAdcVlyDAdcFaild : Inport  RequirementInfo={} %GIDa_a9ef4412_4995_4ff8_a712_a0004978e7c0  Port=10
  MotCtrlMotCurrAdcVlyEAdcFaild : Inport  RequirementInfo={} %GIDa_8c5e2e43_d825_49af_8c14_bb63c0e12ba2  Port=11
  MotCtrlMotCurrAdcVlyFAdcFaild : Inport  RequirementInfo={} %GIDa_7ba5334c_0964_494c_9a84_9ee8fa4a837c  Port=12
  MotCtrlDiagcStsIvtr1Inactv : Inport  Port=13
  MotCtrlDiagcStsIvtr2Inactv : Inport  Port=14
  BrdgVltg : Inport  Port=15
  MotCtrlEcuTFild : Inport  RequirementInfo={} %GIDa_37deaa24_f58f_4dab_941a_680d37588f61  Port=16
  MotCtrlMotAgElec : Inport  Port=17
  MotCtrlMotElecMeclPolarity : Inport  Port=18
  MotCtrlMotVelMrf : Inport  Port=19
  MotCtrlPhaOnTiA : Inport  Port=20
  MotCtrlPhaOnTiB : Inport  Port=21
  MotCtrlPhaOnTiC : Inport  Port=22
  MotCtrlPwmPerd : Inport  Port=23
  MotCtrlSysSt : Inport  Port=24
  MotCurrOffsDeltaA : Inport  Port=25
  MotCurrOffsDeltaB : Inport  Port=26
  MotCurrOffsDeltaC : Inport  Port=27
  MotCurrOffsDeltaD : Inport  Port=28
  MotCurrOffsDeltaE : Inport  Port=29
  MotCurrOffsDeltaF : Inport  Port=30
  " MotCtrlCurrMeasWrmIninTestCmplPrev" : Inport  Port=31
  Trigger : TriggerPort  TriggerType=function-call  PortDimensions=1
  Chart1 : Stateflow chart  RequirementInfo={} %GIDa_9666b06e_9e22_4012_a59d_551b4af1f380  TreatAsAtomicUnit=on
  Constant18 : Constant  Value=ELECGLBPRM_IVTRCNT_CNT_U08
  Constant2 : Constant  Value=MAXCURRCORRD_AMPR_F32
  Constant4 : Constant  Value=CurrMeasMinRqrdPhaOnTi
  Constant5 : Constant  Value=CurrMeasEolOffsLoCmuOffs
  Constant6 : Constant  Value=CurrMeasMotAgCompuDly
  CopyRight2 : Subsystem  Description=|  mask(Copyright Information){none=on}
      | Copyright info block.                                               
      |                                                                     
      | Place copyright information at the top of every subsystem in design.
      mask prompts: none "No parameters"
      mask help: Place copyright information at the top of every subsystem in design.
      mask Display:
      | NxtrConf = 'Nexteer Confidential';
      | 
      | sys = bdroot; %handle for the current model ("system")
      | first = get_param(sys,'Created');
      | first = first(end-3:end);  %year is last four digits
      | 
      | last = get_param(sys,'LastModifiedDate');
      | if isempty(last)
      |     last = datestr(now,'yyyy');
      | else
      |     last = last(end-3:end);
      | end
      | 
      | if strcmp(first,last)
      |     fprintf('%s -- Copyright %s Nexteer',NxtrConf,first)
      | else
      |     fprintf('%s -- %s%s- %s Nexteer',NxtrConf,char(169),first,last)
      | end
  FLTINJ_CURRMEAS_MOTCURRCORRDA1 : Constant  Value=FLTINJ_CURRMEAS_MOTCURRCORRDD
  FltInj_f32 : Subsystem  RequirementInfo={'linktype_rmi_doors' '000089bc (/ESG Group/FDD Module Requirements/EA4 Specific/ES200A_CurrMeas)' '#ES200A_267' 'true' 'REQ: ES200A_267' '' } %GIDa_347b8ae7_8767_40c8_a00c_71aafa320d2d  TreatAsAtomicUnit=on  VariantControl=FltInj_sim  mask(Fault_Injection){}
      mask help: Fault Injection is a simulation only block for EA3 programs.
  MotCurrEolGainA : DataStoreRead  DataStoreName=MotCurrEolGainA
  MotCurrEolGainB : DataStoreRead  DataStoreName=MotCurrEolGainB
  MotCurrEolGainC : DataStoreRead  DataStoreName=MotCurrEolGainC
  MotCurrEolGainD : DataStoreRead  DataStoreName=MotCurrEolGainD
  MotCurrEolGainE : DataStoreRead  DataStoreName=MotCurrEolGainE
  MotCurrEolGainF : DataStoreRead  DataStoreName=MotCurrEolGainF
  MotCurrOffsLoAvrgA : DataStoreRead  DataStoreName=MotCurrOffsLoAvrgA
  MotCurrOffsLoAvrgB : DataStoreRead  DataStoreName=MotCurrOffsLoAvrgB
  MotCurrOffsLoAvrgC : DataStoreRead  DataStoreName=MotCurrOffsLoAvrgC
  MotCurrOffsLoAvrgD : DataStoreRead  DataStoreName=MotCurrOffsLoAvrgD
  MotCurrOffsLoAvrgE : DataStoreRead  DataStoreName=MotCurrOffsLoAvrgE
  MotCurrOffsLoAvrgF : DataStoreRead  DataStoreName=MotCurrOffsLoAvrgF
  Saturation Dynamic1 : simulink/Discontinuities/Saturation Dynamic  RequirementInfo={} %GIDa_a678ac9c_94e0_45a6_bd24_feb3ddad182c  OutMin=[]  OutMax=[]  OutDataTypeStr=Inherit: Same as second input  OutDataType=fixdt(1, 16)  OutScaling=2^-10  DoSatur=off
  Saturation Dynamic2 : simulink/Discontinuities/Saturation Dynamic  RequirementInfo={} %GIDa_ad27d5c1_4180_4794_bb6c_e90600e03b36  OutMin=[]  OutMax=[]  OutDataTypeStr=Inherit: Same as second input  OutDataType=fixdt(1, 16)  OutScaling=2^-10  DoSatur=off
  Saturation Dynamic3 : simulink/Discontinuities/Saturation Dynamic  RequirementInfo={} %GIDa_b6946fe3_e777_41d1_91e9_ba0e49afc616  OutMin=[]  OutMax=[]  OutDataTypeStr=Inherit: Same as second input  OutDataType=fixdt(1, 16)  OutScaling=2^-10  DoSatur=off
  Saturation Dynamic4 : simulink/Discontinuities/Saturation Dynamic  RequirementInfo={} %GIDa_eac887ff_7631_462d_b878_5019172b3d55  OutMin=[]  OutMax=[]  OutDataTypeStr=Inherit: Same as second input  OutDataType=fixdt(1, 16)  OutScaling=2^-10  DoSatur=off
  Saturation Dynamic5 : simulink/Discontinuities/Saturation Dynamic  RequirementInfo={} %GIDa_d9181953_bf05_4f89_9278_4fcbc01ab15c  OutMin=[]  OutMax=[]  OutDataTypeStr=Inherit: Same as second input  OutDataType=fixdt(1, 16)  OutScaling=2^-10  DoSatur=off
  Saturation Dynamic6 : simulink/Discontinuities/Saturation Dynamic  RequirementInfo={} %GIDa_4da0401d_6120_4b21_aef3_0a502043331b  OutMin=[]  OutMax=[]  OutDataTypeStr=Inherit: Same as second input  OutDataType=fixdt(1, 16)  OutScaling=2^-10  DoSatur=off
  Terminator : Terminator
  Unary Minus : UnaryMinus
  Unit Delay1 : UnitDelay  SampleTime=-1  StateName=MotCurrRollgCnt2Prev  StateMustResolveToSignalObject=on
      settings: AttributesFormatString=|
      | State Variable:
      | %<StateName>
  Unit Delay2 : UnitDelay  SampleTime=-1  StateName=MotCurrRollgCnt1Prev  StateMustResolveToSignalObject=on
      settings: AttributesFormatString=|
      | State Variable:
      | %<StateName>
  Unit Delay3 : UnitDelay  SampleTime=-1  StateName=MotCtrlNtc5DErrCntPrev  StateMustResolveToSignalObject=on
      settings: AttributesFormatString=|
      | State Variable:
      | %<StateName>
  Unit Delay4 : UnitDelay  SampleTime=-1  StateName=MotCtrlNtc6DErrCntPrev  StateMustResolveToSignalObject=on
      settings: AttributesFormatString=|
      | State Variable:
      | %<StateName>
  Unit Delay5 : UnitDelay  SampleTime=-1  StateName=PhaOnTiErrCntPrev  StateMustResolveToSignalObject=on
      settings: AttributesFormatString=|
      | State Variable:
      | %<StateName>
  MotCtrlMotCurrCorrdA : Outport  RequirementInfo={} %GIDa_be45cc68_c253_4805_9e57_9f0cd86a4b75
  MotCtrlMotCurrCorrdB : Outport  RequirementInfo={} %GIDa_38a03b4c_0b98_4645_8602_2d424e547661  Port=2
  MotCtrlMotCurrCorrdC : Outport  RequirementInfo={} %GIDa_14a10ace_ee81_4ce4_9336_8f01f385929c  Port=3
  MotCtrlMotCurrCorrdD : Outport  RequirementInfo={} %GIDa_2faaf7ab_4344_43ac_a199_98727489f260  Port=4
  MotCtrlMotCurrCorrdE : Outport  RequirementInfo={} %GIDa_8650b4b3_021a_4514_9f56_5151faf8a566  Port=5
  MotCtrlMotCurrCorrdF : Outport  RequirementInfo={} %GIDa_2593a86b_f65b_45be_b765_d74bea967e23  Port=6
  MotCtrlCurrMeasMotAgCorrd : Outport  RequirementInfo={} %GIDa_90a95302_1bff_47e7_a89a_896fae3a575d  Port=7
  MotCtrlMotCurrRollgCntr1 : Outport  RequirementInfo={} %GIDa_aefa170b_455b_48cb_95aa_73c7254f08bd  Port=8
  MotCtrlMotCurrRollgCntr2 : Outport  RequirementInfo={} %GIDa_b45ba8e0_1343_4e05_96b1_238e41ca7131  Port=9
  MotCtrlNtc5DErrCnt : Outport  RequirementInfo={} %GIDa_6d95d8c9_c06f_4998_9e76_5195a73bd44f  Port=10
  MotCtrlNtc6DErrCnt : Outport  RequirementInfo={} %GIDa_f3d2e981_43dc_4e53_81d4_c9088f8342fd  Port=11
  wires:
  MotCtrlEcuTFild/1 -> Terminator/1
  MotCtrlMotCurrAdcVlyAAdcFaild/1 -> Chart1/7(MotCtrlMotCurrAdcVlyAAdcFaild)
  MotCtrlMotCurrAdcVlyBAdcFaild/1 -> Chart1/8(MotCtrlMotCurrAdcVlyBAdcFaild)
  MotCtrlMotCurrAdcVlyDAdcFaild/1 -> Chart1/10(MotCtrlMotCurrAdcVlyDAdcFaild)
  MotCtrlMotCurrAdcVlyFAdcFaild/1 -> Chart1/12(MotCtrlMotCurrAdcVlyFAdcFaild)
  MotCtrlMotCurrAdcVlyEAdcFaild/1 -> Chart1/11(MotCtrlMotCurrAdcVlyEAdcFaild)
  MotCtrlMotCurrAdcVlyCAdcFaild/1 -> Chart1/9(MotCtrlMotCurrAdcVlyCAdcFaild)
  Saturation Dynamic1/1 -> MotCtrlMotCurrCorrdA/1
  FltInj_f32/1(Signal_Out) -> MotCtrlMotCurrCorrdD/1
  FLTINJ_CURRMEAS_MOTCURRCORRDA1/1 -> FltInj_f32/2(Constant)
  Constant4/1 -> Chart1/14(CurrMeasMinRqrdPhaOnTi)
  Constant5/1 -> Chart1/13(CurrMeasEolOffsLoCmuOffs)
  Constant6/1 -> Chart1/15(CurrMeasMotAgCompuDly)
  MotCtrlMotVelMrf/1 -> Chart1/21(MotCtrlMotVelMrf)
  MotCtrlMotElecMeclPolarity/1 -> Chart1/20(MotCtrlMotElecMeclPolarity)
  BrdgVltg/1 -> Chart1/16(MotCtrlBrdgVltg)
  MotCtrlDiagcStsIvtr1Inactv/1 -> Chart1/17(MotCtrlDiagcStsIvtr1Inactv)
  MotCtrlDiagcStsIvtr2Inactv/1 -> Chart1/18(MotCtrlDiagcStsIvtr2Inactv)
  Constant18/1 -> Chart1/45(ELECGLBPRM_IVTRCNT_CNT_U08)
  Unit Delay1/1 -> Chart1/50(MotCurrRollgCnt2Prev)
  Unit Delay2/1 -> Chart1/49(MotCurrRollgCnt1Prev)
  Saturation Dynamic4/1 -> FltInj_f32/1(Signal_In)
  Saturation Dynamic2/1 -> MotCtrlMotCurrCorrdB/1
  Saturation Dynamic3/1 -> MotCtrlMotCurrCorrdC/1
  Saturation Dynamic5/1 -> MotCtrlMotCurrCorrdE/1
  Saturation Dynamic6/1 -> MotCtrlMotCurrCorrdF/1
  Chart1/10(MotCtrlMotCurrRollgCntr1) -> MotCtrlMotCurrRollgCntr1/1, Unit Delay2/1
  Chart1/11(MotCtrlMotCurrRollgCntr2) -> MotCtrlMotCurrRollgCntr2/1, Unit Delay1/1
  Chart1/1(MotCtrlCurrMeasMotAgCorrd) -> MotCtrlCurrMeasMotAgCorrd/1
  MotCurrOffsLoAvrgB/1 -> Chart1/40(MotCurrOffsLoAvrgB)
  MotCurrOffsLoAvrgA/1 -> Chart1/39(MotCurrOffsLoAvrgA)
  MotCurrOffsLoAvrgD/1 -> Chart1/42(MotCurrOffsLoAvrgD)
  MotCurrOffsLoAvrgC/1 -> Chart1/41(MotCurrOffsLoAvrgC)
  MotCurrOffsLoAvrgF/1 -> Chart1/44(MotCurrOffsLoAvrgF)
  MotCurrOffsLoAvrgE/1 -> Chart1/43(MotCurrOffsLoAvrgE)
  MotCurrEolGainF/1 -> Chart1/32(MotCurrEolGainF)
  MotCurrEolGainD/1 -> Chart1/30(MotCurrEolGainD)
  MotCurrEolGainE/1 -> Chart1/31(MotCurrEolGainE)
  MotCurrEolGainB/1 -> Chart1/28(MotCurrEolGainB)
  MotCurrEolGainC/1 -> Chart1/29(MotCurrEolGainC)
  MotCurrEolGainA/1 -> Chart1/27(MotCurrEolGainA)
  MotCurrOffsDeltaD/1 -> Chart1/36(MotCurrOffsDeltaD)
  MotCurrOffsDeltaC/1 -> Chart1/35(MotCurrOffsDeltaC)
  MotCtrlPhaOnTiC/1 -> Chart1/24(MotCtrlPhaOnTiC)
  MotCtrlSysSt/1 -> Chart1/26(MotCtrlSysSt)
  MotCtrlPwmPerd/1 -> Chart1/25(MotCtrlPwmPerd)
  MotCtrlPhaOnTiB/1 -> Chart1/23(MotCtrlPhaOnTiB)
  MotCurrOffsDeltaE/1 -> Chart1/37(MotCurrOffsDeltaE)
  MotCtrlPhaOnTiA/1 -> Chart1/22(MotCtrlPhaOnTiA)
  MotCurrOffsDeltaF/1 -> Chart1/38(MotCurrOffsDeltaF)
  MotCurrOffsDeltaA/1 -> Chart1/33(MotCurrOffsDeltaA)
  MotCurrOffsDeltaB/1 -> Chart1/34(MotCurrOffsDeltaB)
  Unit Delay4/1 -> Chart1/48(MotCtrlNtc6DErrCntPrev)
  Unit Delay3/1 -> Chart1/47(MotCtrlNtc5DErrCntPrev)
  Chart1/9(MotCtrlNtc6DErrCnt) -> MotCtrlNtc6DErrCnt/1, Unit Delay4/1
  Chart1/8(MotCtrlNtc5DErrCnt) -> MotCtrlNtc5DErrCnt/1, Unit Delay3/1
  " MotCtrlCurrMeasWrmIninTestCmplPrev"/1 -> Chart1/46(MotCtrlCurrMeasWrmIninTestCmplPrev)
  Unit Delay5/1 -> Chart1/51(CurrMeasPhaOnTiErrCntPrev)
  Chart1/12(CurrMeasPhaOnTiErrCnt) -> Unit Delay5/1
  Constant2/1 -> Saturation Dynamic3/1, Saturation Dynamic6/1, Saturation Dynamic5/1, Saturation Dynamic4/1, Saturation Dynamic2/1, Saturation Dynamic1/1, Unary Minus/1
  Unary Minus/1 -> Saturation Dynamic3/3, Saturation Dynamic6/3, Saturation Dynamic5/3, Saturation Dynamic4/3, Saturation Dynamic2/3, Saturation Dynamic1/3
  Chart1/2(MotCtrlMotCurrCorrdA) -> Saturation Dynamic1/2
  Chart1/3(MotCtrlMotCurrCorrdB) -> Saturation Dynamic2/2
  Chart1/4(MotCtrlMotCurrCorrdC) -> Saturation Dynamic3/2
  Chart1/5(MotCtrlMotCurrCorrdD) -> Saturation Dynamic4/2
  Chart1/6(MotCtrlMotCurrCorrdE) -> Saturation Dynamic5/2
  Chart1/7(MotCtrlMotCurrCorrdF) -> Saturation Dynamic6/2
  MotCtrlMotAgElec/1 -> Chart1/19(MotCtrlMotAgElec)
  MotCtrlMotCurrAdcVlyE/1 -> Chart1/5(MotCtrlMotCurrAdcVlyE)
  MotCtrlMotCurrAdcVlyD/1 -> Chart1/4(MotCtrlMotCurrAdcVlyD)
  MotCtrlMotCurrAdcVlyB/1 -> Chart1/2(MotCtrlMotCurrAdcVlyB)
  MotCtrlMotCurrAdcVlyC/1 -> Chart1/3(MotCtrlMotCurrAdcVlyC)
  MotCtrlMotCurrAdcVlyF/1 -> Chart1/6(MotCtrlMotCurrAdcVlyF)
  MotCtrlMotCurrAdcVlyA/1 -> Chart1/1(MotCtrlMotCurrAdcVlyA)

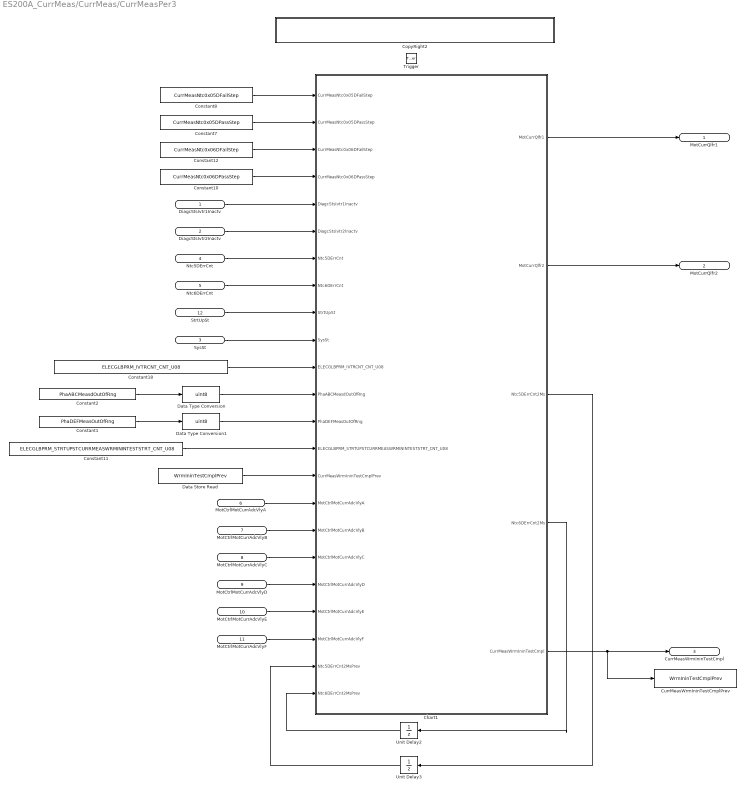
== system ES200A_CurrMeas/CurrMeas/CurrMeasPer3 ==
  DiagcStsIvtr1Inactv : Inport  RequirementInfo={} %GIDa_3f2b24ca_5e64_4642_910e_ca50d78da245
  DiagcStsIvtr2Inactv : Inport  RequirementInfo={} %GIDa_b1a5f59d_5a54_42de_8529_fc0d027b3ef3  Port=2
  SysSt : Inport  RequirementInfo={} %GIDa_ebc52ed6_1f51_43d3_a6da_39b6b9940c04  Port=3  OutDataTypeStr=single
  Ntc5DErrCnt : Inport  RequirementInfo={} %GIDa_ffc53944_d65d_4434_9c9b_5bfc70525927  Port=4  OutDataTypeStr=uint16
  Ntc6DErrCnt : Inport  RequirementInfo={} %GIDa_365cbd76_0dca_48e8_96f7_4dd33cc79fcb  Port=5  OutDataTypeStr=uint16
  MotCtrlMotCurrAdcVlyA : Inport  RequirementInfo={} %GIDa_7bf3cbd7_2538_4e8a_a22d_abe526b19335  Port=6
  MotCtrlMotCurrAdcVlyB : Inport  RequirementInfo={} %GIDa_7698553c_2590_423a_a37b_077079574e3f  Port=7
  MotCtrlMotCurrAdcVlyC : Inport  RequirementInfo={} %GIDa_493e93c2_e8a9_4c58_98a0_ce115796497b  Port=8
  MotCtrlMotCurrAdcVlyD : Inport  RequirementInfo={} %GIDa_dcf6e783_ea97_45aa_b2df_a8b40ffd71d9  Port=9
  MotCtrlMotCurrAdcVlyE : Inport  RequirementInfo={} %GIDa_a4c14b22_ad3d_4d49_8f67_e25589a32bce  Port=10
  MotCtrlMotCurrAdcVlyF : Inport  RequirementInfo={} %GIDa_1f7c68b9_6400_46f6_8cd6_6a391c1de49a  Port=11
  StrtUpSt : Inport  RequirementInfo={} %GIDa_1f30c06a_d58b_4090_b4a6_84109da18cdc  Port=12  OutDataTypeStr=single
  Trigger : TriggerPort  TriggerType=function-call  PortDimensions=1
  Chart1 : Stateflow chart  TreatAsAtomicUnit=on
  Constant1 : Constant  Value=PhaDEFMeasOutOfRng
  Constant10 : Constant  Value=CurrMeasNtc0x06DPassStep
  Constant11 : Constant  Value=ELECGLBPRM_STRTUPSTCURRMEASWRMININTESTSTRT_CNT_U08
  Constant12 : Constant  Value=CurrMeasNtc0x06DFailStep
  Constant18 : Constant  Value=ELECGLBPRM_IVTRCNT_CNT_U08
  Constant2 : Constant  Value=PhaABCMeasdOutOfRng
  Constant7 : Constant  Value=CurrMeasNtc0x05DPassStep
  Constant8 : Constant  Value=CurrMeasNtc0x05DFailStep
  CopyRight2 : Subsystem  Description=|  mask(Copyright Information){none=on}
      | Copyright info block.                                               
      |                                                                     
      | Place copyright information at the top of every subsystem in design.
      mask prompts: none "No parameters"
      mask help: Place copyright information at the top of every subsystem in design.
      mask Display:
      | NxtrConf = 'Nexteer Confidential';
      | 
      | sys = bdroot; %handle for the current model ("system")
      | first = get_param(sys,'Created');
      | first = first(end-3:end);  %year is last four digits
      | 
      | last = get_param(sys,'LastModifiedDate');
      | if isempty(last)
      |     last = datestr(now,'yyyy');
      | else
      |     last = last(end-3:end);
      | end
      | 
      | if strcmp(first,last)
      |     fprintf('%s -- Copyright %s Nexteer',NxtrConf,first)
      | else
      |     fprintf('%s -- %s%s- %s Nexteer',NxtrConf,char(169),first,last)
      | end
  CurrMeasWrmIninTestCmplPrev : DataStoreWrite  RequirementInfo={} %GIDa_56301e73_d1a5_44f0_9c00_c95c5be8192d  DataStoreName=WrmIninTestCmplPrev  DataStoreElements=WrmIninTestCmplPrev
  Data Store Read : DataStoreRead  DataStoreName=WrmIninTestCmplPrev  DataStoreElements=WrmIninTestCmplPrev
  Data Type Conversion : DataTypeConversion  OutDataTypeStr=uint8
  Data Type Conversion1 : DataTypeConversion  OutDataTypeStr=uint8
  Unit Delay2 : UnitDelay  SampleTime=-1  StateName=Ntc6DErrCnt2MilliSecPrev  StateMustResolveToSignalObject=on
      settings: AttributesFormatString=|
      | State Variable:
      | %<StateName>
  Unit Delay3 : UnitDelay  SampleTime=-1  StateName=Ntc5DErrCnt2MilliSecPrev  StateMustResolveToSignalObject=on
      settings: AttributesFormatString=|
      | State Variable:
      | %<StateName>
  MotCurrQlfr1 : Outport  RequirementInfo={} %GIDa_97d5bfb1_2351_42dd_b658_023a6d8f5aa1
  MotCurrQlfr2 : Outport  RequirementInfo={} %GIDa_e2da2e04_5849_4da3_a687_01333d2236a2  Port=2
  CurrMeasWrmIninTestCmpl : Outport  RequirementInfo={} %GIDa_b01ce9a2_2e51_43fa_ab76_6aeab0dbecf7  Port=3
  wires:
  Constant10/1 -> Chart1/4(CurrMeasNtc0x06DPassStep)
  Constant7/1 -> Chart1/2(CurrMeasNtc0x05DPassStep)
  Constant12/1 -> Chart1/3(CurrMeasNtc0x06DFailStep)
  Constant8/1 -> Chart1/1(CurrMeasNtc0x05DFailStep)
  DiagcStsIvtr1Inactv/1 -> Chart1/5(DiagcStsIvtr1Inactv)
  DiagcStsIvtr2Inactv/1 -> Chart1/6(DiagcStsIvtr2Inactv)
  Ntc5DErrCnt/1 -> Chart1/7(Ntc5DErrCnt)
  Ntc6DErrCnt/1 -> Chart1/8(Ntc6DErrCnt)
  Constant18/1 -> Chart1/11(ELECGLBPRM_IVTRCNT_CNT_U08)
  Constant11/1 -> Chart1/14(ELECGLBPRM_STRTUPSTCURRMEASWRMININTESTSTRT_CNT_U08)
  SysSt/1 -> Chart1/10(SysSt)
  Chart1/3(Ntc5DErrCnt2Ms) -> Unit Delay3/1
  Chart1/4(Ntc6DErrCnt2Ms) -> Unit Delay2/1
  Chart1/5(CurrMeasWrmIninTestCmpl) -> CurrMeasWrmIninTestCmpl/1, CurrMeasWrmIninTestCmplPrev/1
  Chart1/1(MotCurrQlfr1) -> MotCurrQlfr1/1
  Chart1/2(MotCurrQlfr2) -> MotCurrQlfr2/1
  Unit Delay2/1 -> Chart1/23(Ntc6DErrCnt2MsPrev)
  Unit Delay3/1 -> Chart1/22(Ntc5DErrCnt2MsPrev)
  Data Store Read/1 -> Chart1/15(CurrMeasWrmIninTestCmplPrev)
  Constant1/1 -> Data Type Conversion1/1
  Constant2/1 -> Data Type Conversion/1
  Data Type Conversion/1 -> Chart1/12(PhaABCMeasdOutOfRng)
  Data Type Conversion1/1 -> Chart1/13(PhaDEFMeasOutOfRng)
  MotCtrlMotCurrAdcVlyA/1 -> Chart1/16(MotCtrlMotCurrAdcVlyA)
  MotCtrlMotCurrAdcVlyB/1 -> Chart1/17(MotCtrlMotCurrAdcVlyB)
  MotCtrlMotCurrAdcVlyC/1 -> Chart1/18(MotCtrlMotCurrAdcVlyC)
  MotCtrlMotCurrAdcVlyD/1 -> Chart1/19(MotCtrlMotCurrAdcVlyD)
  MotCtrlMotCurrAdcVlyE/1 -> Chart1/20(MotCtrlMotCurrAdcVlyE)
  MotCtrlMotCurrAdcVlyF/1 -> Chart1/21(MotCtrlMotCurrAdcVlyF)
  StrtUpSt/1 -> Chart1/9(StrtUpSt)

== system ES200A_CurrMeas/CurrMeas/FltInj_f32 ==
  note: This block requires no modification by FDD author.
      |
      | This block does not actually simulate any fault injection.  It is simply a pass-thru.
      |
      | The Constant port (#2) simply terminates its signal, but we are trying to force the FDD author
      | to properly use the FltInjectionLocType enumeration in FDD model.
  note: EA4.x Fault Injection
  Signal_In : Inport
  Constant : Inport  Port=2
  CopyRight2 : Subsystem  Description=|  mask(Copyright Information){none=on}
      | Copyright info block.                                               
      |                                                                     
      | Place copyright information at the top of every subsystem in design.
      mask prompts: none "No parameters"
      mask help: Place copyright information at the top of every subsystem in design.
      mask Display:
      | NxtrConf = 'Nexteer Confidential';
      | 
      | sys = bdroot; %handle for the current model ("system")
      | first = get_param(sys,'Created');
      | first = first(end-3:end);  %year is last four digits
      | 
      | last = get_param(sys,'LastModifiedDate');
      | if isempty(last)
      |     last = datestr(now,'yyyy');
      | else
      |     last = last(end-3:end);
      | end
      | 
      | if strcmp(first,last)
      |     fprintf('%s -- Copyright %s Nexteer',NxtrConf,first)
      | else
      |     fprintf('%s -- %s%s- %s Nexteer',NxtrConf,char(169),first,last)
      | end
  Terminator : Terminator
  Signal_Out : Outport
  wires:
  Signal_In/1 -> Signal_Out/1
  Constant/1 -> Terminator/1

== system ES200A_CurrMeas/CurrMeas/CurrMeasEolGainReq/CopyRight2 ==

== system ES200A_CurrMeas/CurrMeas/CurrMeasEolGainStsReq/CopyRight2 ==

== system ES200A_CurrMeas/CurrMeas/CurrMeasEolOffsReq/CopyRight2 ==

== system ES200A_CurrMeas/CurrMeas/CurrMeasEolOffsStsReq/CopyRight2 ==

== system ES200A_CurrMeas/CurrMeas/CurrMeasGainReadReq/CopyRight2 ==

== system ES200A_CurrMeas/CurrMeas/CurrMeasGainWrReq/CopyRight2 ==

== system ES200A_CurrMeas/CurrMeas/CurrMeasGainWrReq/IF ==
  CurrMeasMotCurrGainA_ArgIn : Inport  RequirementInfo={} %GIDa_87b59b63_6625_4c38_a995_a430fafe0129  OutDataTypeStr=single
  CurrMeasMotCurrGainB_ArgIn : Inport  RequirementInfo={} %GIDa_77d3c118_6d5d_4a6d_bf43_acbab5c55649  Port=2  OutDataTypeStr=single
  CurrMeasMotCurrGainC_ArgIn : Inport  RequirementInfo={} %GIDa_50760476_4eb4_4fe6_81a8_acdf6cdf4679  Port=3  OutDataTypeStr=single
  CurrMeasMotCurrGainD_ArgIn : Inport  RequirementInfo={} %GIDa_e8971956_e66c_49cd_b063_7f3e149dc0e1  Port=4  OutDataTypeStr=single
  CurrMeasMotCurrGainE_ArgIn : Inport  RequirementInfo={} %GIDa_9ee4b377_1ed8_4e03_968c_c6f167646a4a  Port=5  OutDataTypeStr=single
  CurrMeasMotCurrGainF_ArgIn : Inport  RequirementInfo={} %GIDa_824e1cae_8662_42c6_b5bf_076ba0b66ddf  Port=6  OutDataTypeStr=single
  Action Port : ActionPort  ActionType=then
  Constant14 : Constant  OutDataTypeStr=single
  CurrMeasEolGainCalSet : DataStoreWrite  RequirementInfo={'linktype_rmi_doors' '000089bc (/ESG Group/FDD Module Requirements/EA4 Specific/ES200A_CurrMeas)' '#ES200A_291' 'true' 'REQ: ES200A_291' '' } %GIDa_e0bf40b3_7bb6_4054_b3a0_3f5c2964ab0c  DataStoreName=CurrMeasEolGainCalSet  DataStoreElements=CurrMeasEolGainCalSet.CurrMeasMotCurrEolGainA#CurrMeasEolGainCalSet.CurrMeasMotCurrEolGainB#CurrMeasEolGainCalSet.CurrMeasMotCurrEolGainC#CurrMeasEolGainCalSet.CurrMeasMotCurrEolGainD#CurrMeasEolGainCalSet.CurrMeasMotCurrEolGainE#CurrMeasEolGainCalSet.CurrMeasMotCurrEolGainF
  CurrMeasEolGainCalSet_SetRamBlockStatus : Subsystem  RequirementInfo={'linktype_rmi_doors' '000089bc (/ESG Group/FDD Module Requirements/EA4 Specific/ES200A_CurrMeas)' '#ES200A_291' 'true' 'REQ: ES200A_291' '' } %GIDa_5922b5b3_8031_4b5e_94b1_30094195ff33  TreatAsAtomicUnit=on
  Positive Response : Constant  Value=0
  CurrMeasGainWrReqSts : Outport  RequirementInfo={} %GIDa_db75dea6_25d1_4b9e_bf3d_93caa7994694
  wires:
  Constant14/1 -> CurrMeasEolGainCalSet_SetRamBlockStatus/1("BlockChanged ")
  CurrMeasMotCurrGainA_ArgIn/1 -> CurrMeasEolGainCalSet/1
  CurrMeasMotCurrGainB_ArgIn/1 -> CurrMeasEolGainCalSet/2
  CurrMeasMotCurrGainD_ArgIn/1 -> CurrMeasEolGainCalSet/4
  CurrMeasMotCurrGainE_ArgIn/1 -> CurrMeasEolGainCalSet/5
  CurrMeasMotCurrGainC_ArgIn/1 -> CurrMeasEolGainCalSet/3
  CurrMeasMotCurrGainF_ArgIn/1 -> CurrMeasEolGainCalSet/6
  Positive Response/1 -> CurrMeasGainWrReqSts/1

== system ES200A_CurrMeas/CurrMeas/CurrMeasGainWrReq/else  ==
  Action Port : ActionPort  ActionType=else
  Negative Response : Constant
  CurrMeasGainWrReqSts : Outport  RequirementInfo={} %GIDa_7081d4be_b2eb_437d_b738_c85b18ebe99c
  wires:
  Negative Response/1 -> CurrMeasGainWrReqSts/1

== system ES200A_CurrMeas/CurrMeas/CurrMeasInit1/CopyRight2 ==

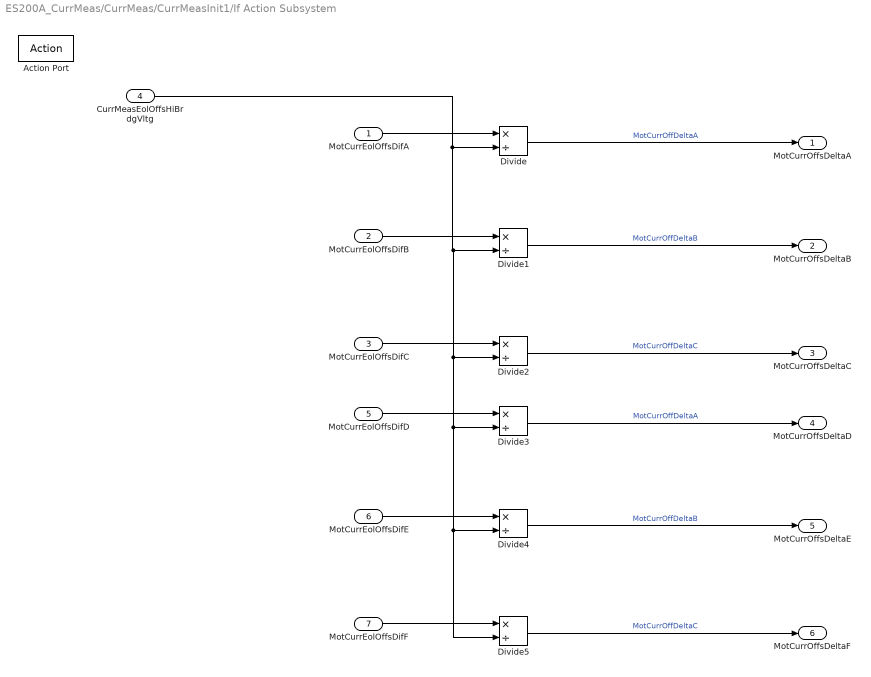
== system ES200A_CurrMeas/CurrMeas/CurrMeasInit1/If Action Subsystem ==
  MotCurrEolOffsDifA : Inport  OutDataTypeStr=single
  MotCurrEolOffsDifB : Inport  Port=2  OutDataTypeStr=single
  MotCurrEolOffsDifC : Inport  Port=3  OutDataTypeStr=single
  CurrMeasEolOffsHiBrdgVltg : Inport  Port=4  OutDataTypeStr=single
  MotCurrEolOffsDifD : Inport  Port=5  OutDataTypeStr=single
  MotCurrEolOffsDifE : Inport  Port=6  OutDataTypeStr=single
  MotCurrEolOffsDifF : Inport  Port=7  OutDataTypeStr=single
  Action Port : ActionPort  ActionType=then
  Divide{,1..5} (6 alike) : Product  Inputs=*/
  MotCurrOffsDeltaA : Outport  OutDataTypeStr=single
  MotCurrOffsDeltaB : Outport  Port=2  OutDataTypeStr=single
  MotCurrOffsDeltaC : Outport  Port=3  OutDataTypeStr=single
  MotCurrOffsDeltaD : Outport  Port=4  OutDataTypeStr=single
  MotCurrOffsDeltaE : Outport  Port=5  OutDataTypeStr=single
  MotCurrOffsDeltaF : Outport  Port=6  OutDataTypeStr=single
  wires:
  MotCurrEolOffsDifA/1 -> Divide/1
  MotCurrEolOffsDifB/1 -> Divide1/1
  MotCurrEolOffsDifC/1 -> Divide2/1
  Divide/1 -> MotCurrOffsDeltaA/1  "MotCurrOffDeltaA"
  Divide1/1 -> MotCurrOffsDeltaB/1  "MotCurrOffDeltaB"
  Divide2/1 -> MotCurrOffsDeltaC/1  "MotCurrOffDeltaC"
  MotCurrEolOffsDifD/1 -> Divide3/1
  MotCurrEolOffsDifE/1 -> Divide4/1
  MotCurrEolOffsDifF/1 -> Divide5/1
  CurrMeasEolOffsHiBrdgVltg/1 -> Divide5/2, Divide4/2, Divide3/2, Divide2/2, Divide1/2, Divide/2
  Divide3/1 -> MotCurrOffsDeltaD/1  "MotCurrOffDeltaA"
  Divide4/1 -> MotCurrOffsDeltaE/1  "MotCurrOffDeltaB"
  Divide5/1 -> MotCurrOffsDeltaF/1  "MotCurrOffDeltaC"
